simulink model "Joystick201401010_method1"  (R2012b)
settings: Solver=ode4  StartTime=0.0  StopTime=inf  FixedStep=sample_time  RelTol=1e-3
InitFcn:
  | sample_time=0.005;%0.004;%0.0025;%0.02;
  | sample_time_Vicon = 0.005;
  | DeltaT = 0.02;
  | g = 9.81;
  | H0 = g%0.3165;
  | Kl = 1;
  | 
  | Omega_r = 1.31;%for Horizontal reference
  | Zeta_r = 1; %for Horizontal reference
  | Omega = 1.31;%for Horizontal Control
  | Zeta = 0.7;    %for Horizontal Control
  | 
  | Omega_h_r = 2.2; %for vertical reference
  | Zeta_h_r = 1;  %for vertical reference
  | Omega_h = 2.2;    %for vertical control
  | Zeta_h = 1;         %for vertical control
  | PI=pi;
  | 
  | Mass = 1.1;
  | Acc_Max = 4;
  | Acc_Max_h = 4;
  | 
  | Max_RP = 60;
  | 
  | % for NN
  | n = 5;
  | r = 3;
  | n2 = 5;
  | NN_ST = 0.02;
  | 
  | GAMA_V = 3;
  | gama_V_e = 0.01;
  | 
  | GAMA_W = GAMA_V;
  | gama_W_e =0.01;
  | 
  | % deadzone
  | NN_Deadzone_Z = 0;
  | 
  | % inputs nomalizaton parameters
  | NN_Z_y_min = -3;
  | NN_Z_y_max = 0.5;
  | 
  | NN_Z_v_max = 8;
  | NN_Z_v_min = -NN_Z_v_max;
  | 
  | % alpha = 0.034;
  | alpha = 1;
  | % c_f = 0.0015;
  | c_f = 0.001;
  | c_y_tilt = 1*0.5;
  | 
  | %for WK paras
  | Heightcontrol = 0.08;
  | Scale_Factor=1;
  | yoffset=0;
  | 
  | load MaoBi_Oct04_2_int.mat
  | MB_Interp.time = [];
undefined symbols (not defined in the file or in its folder): DiscIntNeverNeededParam
libraries: simulink x10, X330_Control x4, vrlib x1
(part 2 of 2)

== stateflow chart Joystick201401010_method1/Planning/Trajectory Logic/UAV SF ==
  note: Joystick[x]:
      |
      | 0. X-axis
      | 1. Y-axis
      | 2. Z-Axis
      | 3. PWM
      |
      | Joystick Trigger = Trigger state
      |
      |
      | TooClose[x]:
      |
      | Where x=:
      | 0.	Bound
      | 1.	Q5 Current Radius
      | 2.	X
      | 3.	Y
  state AirBorne
    state Game
      state InZone
        state MovetoCenter
          en:
          PosDesired [0]	= 0;
          PosDesired [1]	= 0;
        state Descent3
          en:PosDesired [2]	= -0.98;
        state Resumeback2
          en:
          ClawDone = 2;
        state Descent
          en:
          PosDesired [2] = -0.86;
          PosDesired [0]	= 0;
          PosDesired [1]	= 0;
        state CloseClaw1
          en:
          PWM = 1200;
        state Ascent1
          en:
          PosDesired [2]	 = Joystick[2];
        (default) -> Descent3 : {PWM			= 1690;
            | LightPWM		= 1650;}
        Descent3 -> Descent : after (1.3,sec)
        MovetoCenter -> Descent : [(abs(Pos[0]-PosDesired[0])+abs(Pos[1]-PosDesired[1]))<0.02]
        Ascent1 -> Resumeback2 : [abs(Pos[2]-PosDesired[2])<0.03]
        Descent -> CloseClaw1 : [abs(Pos[2]-PosDesired [2])<0.02]
        CloseClaw1 -> Ascent1 : after (0.7,sec)
      state JoystickCon
        du: PosDesired [0]  	= Joystick[0];
        PosDesired [1]	= Joystick[1];
        PosDesired [2]  	= Joystick[2];
        PWM 			= Joystick[3];
        LightPWM		= 1450;
      state ResetJoyStick1
        en:
        ClawDone = 0;
        JoystickReset	= 0;
      state Flyaway
        en:
        XFly 			= TooClose[2];
        YFly 			= TooClose[3];
        LightPWM 		= 1250;
        JoystickReset 	= 1;
      state Fly
        du:
        PosDesired[0] = (XFly-PosDesired[0])*1.7*DeltaT + PosDesired[0];
        PosDesired[1] = (YFly-PosDesired[1])*1.7*DeltaT + PosDesired[1];
      InZone -> ResetJoyStick1 : [ClawDone ==2]
      JoystickCon -> InZone [order 1] : [(TooClose[1]<=0.6)&&(JoystickTrigger==1)]
      (default) -> ResetJoyStick1
      ResetJoyStick1 -> JoystickCon
      Fly -> ResetJoyStick1 : after (2.3,sec)
      JoystickCon -> Flyaway [order 2] : [TooClose[0]==2]
      Flyaway -> Fly
    state TakeOff
      du:HoverThrottle = (H0 - HoverThrottle)*3*DeltaT + HoverThrottle ;
      PosDesired[2]  = (-1.2- PosDesired[2])*1*DeltaT + PosDesired[2] ;
    state ResetJoyStick
      en:
      JoystickReset = 1;
      PosDesired [3] = 0;
    state Safety
      state HoverXY
        en:
        PosDesired 	= Pos;
        PWM 			= 1690;
        LightPWM 		= 1550;
      state HoverZ
        du:PosDesired[2] = (-1.1-PosDesired[2])*2*DeltaT + PosDesired[2];
      state OffloadPos
        du:
        PosDesired[0] = (-1-PosDesired[0])*0.2*DeltaT + PosDesired[0];
        PosDesired[1] = (3.3-PosDesired[1])*0.2*DeltaT + PosDesired[1];
      state Descent2
        du: PosDesired[2] = (-0.57-PosDesired[2])*3*DeltaT + PosDesired[2];
      (default) -> HoverXY
      HoverXY -> HoverZ : [Q4[2]<-2]
      HoverZ -> OffloadPos : [abs(Pos[2]+1.1)<0.02]
      OffloadPos -> Descent2 : [(abs(Pos[0]+1)+abs(Pos[1]-3.3))<0.3]
    (default) -> TakeOff : {PosDesired = Pos;}
    ResetJoyStick -> Game
    TakeOff -> ResetJoyStick [order 2] : [(abs(Q4[0]+2)+abs(Q4[1]))<0.2]
    TakeOff -> ResetJoyStick [order 1] : after (3,sec)
    Game -> Safety : [RC[5] > 0]
  state Landing
    state Descending
      en:PosDesired = Pos;
      du:PosDesired[2] = (0.2- PosDesired[2])*0.5*DeltaT + PosDesired[2] ;
    state CutThrottle
      en: PWM=1600;
      du:HoverThrottle = (0.0- HoverThrottle)*3*DeltaT + HoverThrottle ;
    (default) -> Descending : {LightPWM = 1550;}
    Descending -> CutThrottle : [Pos[2] >(0.0 -0.2)]
  Landing -> AirBorne : [RC[6] > 0.5]
  AirBorne -> Landing : [RC[6] < -0.5]
  (default) -> Landing : {HoverThrottle = 0;}
  data: PosDesired output double size=4; HoverThrottle output double size=1; LightPWM output uint16 size=1; RC input size=8; Pos input size=4; DeltaT parameter size=1; H0 parameter size=1; Kl parameter size=1; VelCmd local double size=2 =0; PWM output double; PI parameter size=1; descentrate local double; Joystick input; TooClose input double; JoystickReset output double size=1; XFly local double size=1; YFly local double size=1; ClawDone output double size=1; JoystickTrigger input boolean size=1; Q4 input
